simulink model "actuatorModel"  (R2023b)
settings: Solver=VariableStepAuto  StartTime=0.0  StopTime=Tfinal  RelTol=1e-3
undefined symbols (not defined in the file or in its folder): A, Lw0
settings Model: Creator=kristopherriordan  LastModifiedBy=kristopherriordan

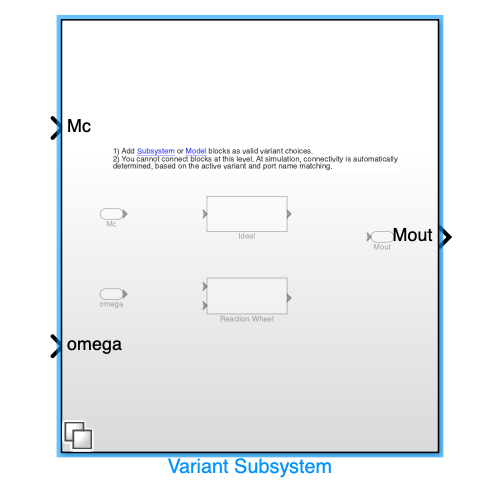
[thumbnail: Simulink's stored preview of the top-level diagram]
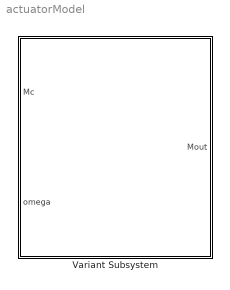
== system actuatorModel ==
  Variant Subsystem : Subsystem  Variant=on

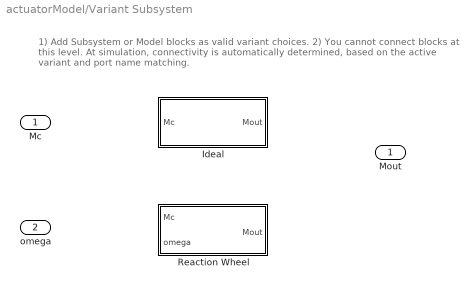
== system actuatorModel/Variant Subsystem ==
  note: 1) Add Subsystem or Model blocks as valid variant choices.
      | 2) You cannot connect blocks at this level. At simulation, connectivity is automatically
      | determined, based on the active variant and port name matching.
  Mc : Inport
  omega : Inport  Port=2
  Ideal : Subsystem  VariantControl="controlMoment==\"ideal\""
  Reaction Wheel : Subsystem  VariantControl="controlMoment==\"reactionWheel\""
  Mout : Outport

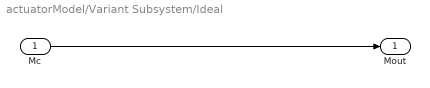
== system actuatorModel/Variant Subsystem/Ideal ==
  Mc : Inport
  Mout : Outport
  wires:
  Mc/1 -> Mout/1

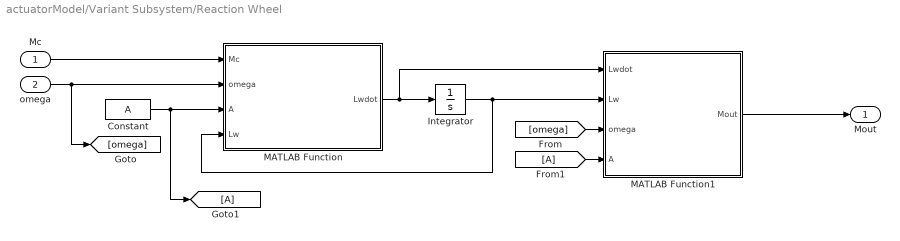
== system actuatorModel/Variant Subsystem/Reaction Wheel ==
  Mc : Inport
  omega : Inport  Port=2
  Constant : Constant  Value=A
  From1 : From
  Goto1 : Goto
  Integrator : Integrator  InitialCondition=Lw0
  MATLAB Function : MATLAB Function  TreatAsAtomicUnit=on
  MATLAB Function1 : MATLAB Function  TreatAsAtomicUnit=on
  Mout : Outport
  wires:
  Mc/1 -> MATLAB Function/1(Mc)
  Constant/1 -> Goto1/1, MATLAB Function/3(A)
  omega/1 -> MATLAB Function/2(omega), [omega]
  MATLAB Function/1(Lwdot) -> MATLAB Function1/1(Lwdot), Integrator/1
  Integrator/1 -> MATLAB Function1/2(Lw), MATLAB Function/4(Lw)
  [omega] -> MATLAB Function1/3(omega)
  From1/1 -> MATLAB Function1/4(A)
  MATLAB Function1/1(Mout) -> Mout/1

== matlab function actuatorModel/Variant Subsystem/Reaction Wheel/MATLAB Function1 ==
  data: Lwdot input; Mout output; Lw input; omega input; A input
function Mout = Lw2Mout(Lwdot, Lw, omega, A)

Mout = -(A * Lwdot) - cross(omega, A * Lw);

== matlab function actuatorModel/Variant Subsystem/Reaction Wheel/MATLAB Function ==
  data: Mc input; Lwdot output; omega input; A input; Lw input
function Lwdot = Mc2Lwdot(Mc, omega, A, Lw)

Lwdot = pinv(A) * (- Mc - cross(omega, A * Lw));
